simulink model "q10"  (R2019a)
settings: Solver=VariableStepAuto  StartTime=0.0  StopTime=0.2  RelTol=1e-3
settings Model: Creator=ADMIN  LastModifiedBy=ADMIN

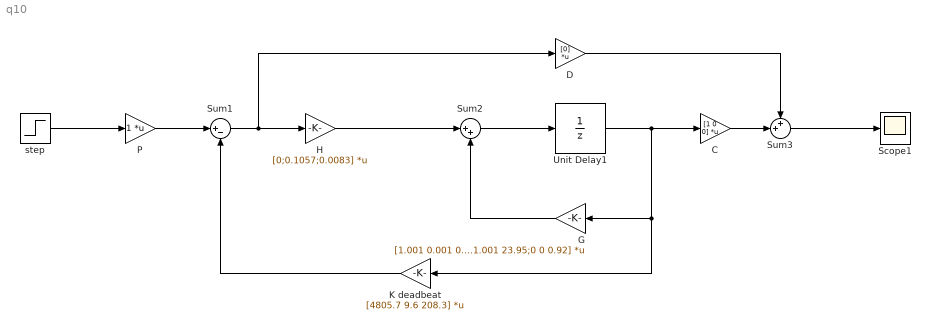
== system q10 ==
  "C " : Gain  Gain=[1 0 0]  Multiplication=Matrix(K*u)
  D : Gain  Gain=[0]  Multiplication=Matrix(K*u)
  G : Gain  Gain=[1.001 0.001 0.012; 1.9 1.001 23.95;0 0 0.92]  Multiplication=Matrix(K*u)
  H : Gain  Gain=[0;0.1057;0.0083]  Multiplication=Matrix(K*u)
  K deadbeat : Gain  Gain=[4805.7 9.6 208.3]  Multiplication=Matrix(K*u)
  P : Gain  Multiplication=Matrix(K*u)
  Scope1 : Scope
  Sum1 : Sum  Inputs=|+-
  Sum2 : Sum  Inputs=|++
  Sum3 : Sum  Inputs=++|
  Unit Delay1 : UnitDelay  SampleTime=0.001  HasFrameUpgradeWarning=on
  step : Step  Time=0  SampleTime=0.001
  wires:
  K deadbeat/1 -> Sum1/2
  P/1 -> Sum1/1
  Sum1/1 -> H/1, D/1
  "C "/1 -> Sum3/2
  G/1 -> Sum2/2
  Unit Delay1/1 -> K deadbeat/1, G/1, "C "/1
  D/1 -> Sum3/1
  Sum2/1 -> Unit Delay1/1
  Sum3/1 -> Scope1/1
  H/1 -> Sum2/1
  step/1 -> P/1
